simulink model "Connectivity"  (R2022a)
settings: Solver=VariableStepAuto  StartTime=0.0  StopTime=10.0  RelTol=1e-3
settings Model: Creator=mariodelossantos  LastModifiedBy=mariodelossantos

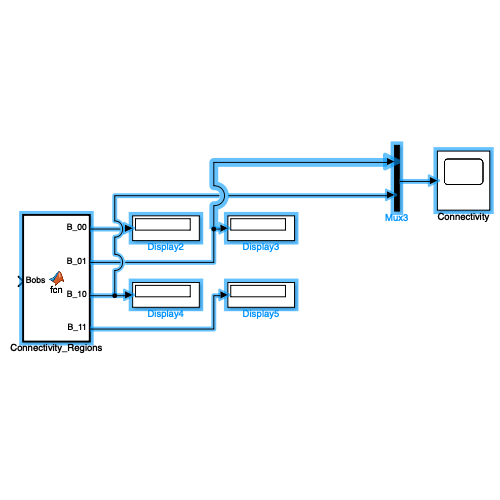
[thumbnail: Simulink's stored preview of the top-level diagram]
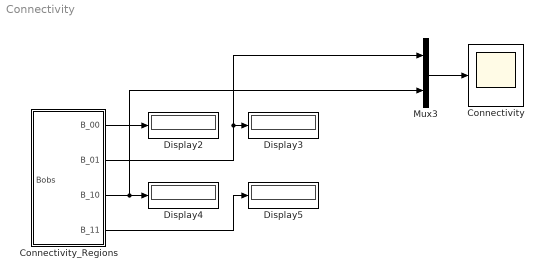
== system Connectivity ==
  Connectivity : Scope
  Connectivity_Regions : MATLAB Function  TreatAsAtomicUnit=on
  Display{2..5} (4 alike) : Display
  Mux3 : Mux  Inputs=2
  wires:
  Connectivity_Regions/4(B_11) -> Display5/1
  Connectivity_Regions/1(B_00) -> Display2/1
  Mux3/1 -> Connectivity/1
  Connectivity_Regions/3(B_10) -> Mux3/2, Display4/1
  Connectivity_Regions/2(B_01) -> Mux3/1, Display3/1

== matlab function Connectivity/Connectivity_Regions ==
  data: Bobs input; B_00 output; B_01 output; B_10 output; B_11 output
function [B_00, B_01, B_10, B_11] = fcn(Bobs)

B_00 = (Bobs(1,1));
B_01 = (Bobs(1,2));
B_10 = (Bobs(2,1));
B_11 = (Bobs(2,2));
